simulink model "PendMod"  (Simulink 8.5)
settings: Solver=ode45  StartTime=0.0  StopTime=tStop  RelTol=1e-3
settings Model: Creator=humphreysb  LastModifiedBy=humphreysb
settings DataIOCC: SignalLoggingSaveFormat=Dataset
settings OptimizationCC: ExpressionDepthLimit=128
settings DebuggingCC: UnderspecifiedInitializationDetection=Simplified  MergeDetectMultiDrivingBlocksExec=error  FcnCallInpInsideContextMsg=EnableAllAsError  StateNameClashWarn=none
settings GRTTargetCC: CombineOutputUpdateFcns=on  GRTInterface=off

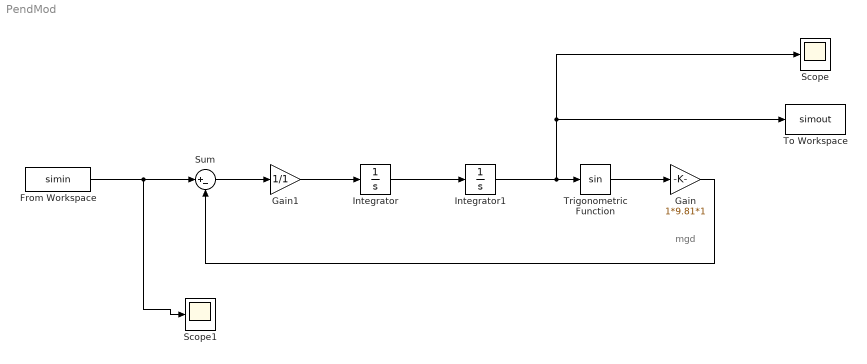
== system PendMod ==
  note: mgd
  From Workspace : FromWorkspace  VariableName=simin  SampleTime=0
  Gain : Gain  Gain=1*9.81*1
  Gain1 : Gain  Gain=1/1
  Integrator : Integrator
  Integrator1 : Integrator
  Scope : Scope
  Scope1 : Scope
  Sum : Sum  Inputs=|+-
  To Workspace : ToWorkspace  VariableName=simout  SampleTime=-1
  Trigonometric Function : Trigonometry
  wires:
  Integrator/1 -> Integrator1/1
  Integrator1/1 -> Scope/1, To Workspace/1, Trigonometric Function/1
  Trigonometric Function/1 -> Gain/1
  Gain1/1 -> Integrator/1
  From Workspace/1 -> Sum/1, Scope1/1
  Sum/1 -> Gain1/1
  Gain/1 -> Sum/2
